simulink model "stateMachineAndGaitPlayback"  (R2016b)
settings: Solver=FixedStepAuto  StartTime=0.0  StopTime=50  FixedStep=0.002  RelTol=1e-3  AbsTol=1e-5
undefined symbols (not defined in the file or in its folder): ExoskeletonState, Leg, StepType
libraries: VariousLibrary x2, simulink x2, GaitHandler x1, StatemachineMARCH x1
settings Model: DataDictionary=ModelDictionary.sldd  Creator=Taeke  LastModifiedBy=Taeke
settings DataIOCC: SaveState=on

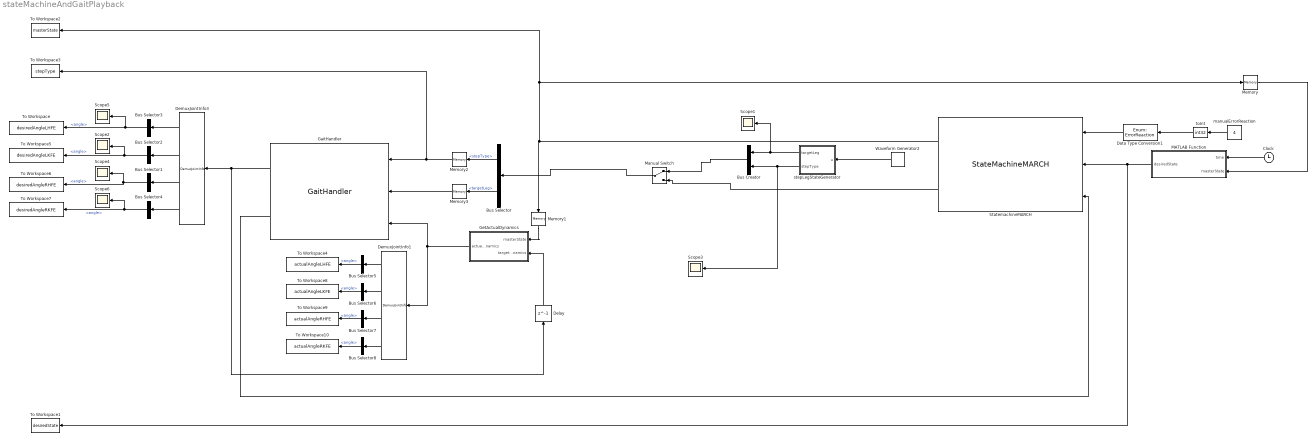
== system stateMachineAndGaitPlayback ==
  Bus Creator : BusCreator  Inputs=2  OutDataTypeStr=Bus: GaitGeneratorInput  NonVirtualBus=on
  Bus Selector : BusSelector  OutputSignals=stepType,targetLeg
  Bus Selector{1..8} (8 alike) : BusSelector  OutputSignals=angle
  Clock : Clock
  Data Type Conversion1 : DataTypeConversion  OutDataTypeStr=Enum: ErrorReaction
  Delay : Delay  DelayLength=1
  DemuxJointInfo1 : VariousLibrary/DemuxJointInfo
  DemuxJointInfo3 : VariousLibrary/DemuxJointInfo
  GaitHandler : GaitHandler/GaitHandler
  GetActualDynamics : Subsystem
  MATLAB Function : MATLAB Function  TreatAsAtomicUnit=on
  Manual Switch : ManualSwitch
  Memory : Memory  X0=ExoskeletonState.MANUAL
  Memory1 : Memory  X0=ExoskeletonState.MANUAL
  Memory2 : Memory  X0=StepType.NOSTEP
  Memory3 : Memory  X0=Leg.NONE
  Scope{1..6} (6 alike) : Scope
  StatemachineMARCH : StatemachineMARCH/StateMachineMARCH
  To Workspace : ToWorkspace  VariableName=desiredAngleLHFE  SaveFormat=Timeseries  SampleTime=-1
  To Workspace1 : ToWorkspace  VariableName=desiredState  SaveFormat=Timeseries  SampleTime=-1
  To Workspace10 : ToWorkspace  VariableName=actualAngleRKFE  SaveFormat=Timeseries  SampleTime=-1
  To Workspace2 : ToWorkspace  VariableName=masterState  SaveFormat=Timeseries  SampleTime=-1
  To Workspace3 : ToWorkspace  VariableName=stepType  SaveFormat=Timeseries  SampleTime=-1
  To Workspace4 : ToWorkspace  VariableName=actualAngleLHFE  SaveFormat=Timeseries  SampleTime=-1
  To Workspace5 : ToWorkspace  VariableName=desiredAngleLKFE  SaveFormat=Timeseries  SampleTime=-1
  To Workspace6 : ToWorkspace  VariableName=desiredAngleRHFE  SaveFormat=Timeseries  SampleTime=-1
  To Workspace7 : ToWorkspace  VariableName=desiredAngleRKFE  SaveFormat=Timeseries  SampleTime=-1
  To Workspace8 : ToWorkspace  VariableName=actualAngleLKFE  SaveFormat=Timeseries  SampleTime=-1
  To Workspace9 : ToWorkspace  VariableName=actualAngleRHFE  SaveFormat=Timeseries  SampleTime=-1
  Waveform Generator2 : simulink/Sources/Waveform Generator  OutMin=[]  OutMax=[]  OutDataTypeStr=double  SelectedSignal=1  Signals=step(1,0,1)+step(8,0,1)+step(9,0,1)+step(10.7,0,1)+step(12.4,0,1)+step(14.1,0,2)-step(15.8,0,5)+step(17,0,6)  BlockNames=MultiportSwitch_7d132669d28647b  SampleTime=-1
  manualErrorReaction : Constant  Value=4
  stepLegStateGenerator : MATLAB Function  TreatAsAtomicUnit=on
  toInt : DataTypeConversion  OutDataTypeStr=int32
  wires:
  Bus Selector/1 -> Memory2/1  "<stepType>"
  Bus Selector/2 -> Memory3/1  "<targetLeg>"
  Memory2/1 -> To Workspace3/1, GaitHandler/1
  Memory3/1 -> GaitHandler/2
  manualErrorReaction/1 -> toInt/1
  toInt/1 -> Data Type Conversion1/1
  Data Type Conversion1/1 -> StatemachineMARCH/1
  GaitHandler/2 -> StatemachineMARCH/3
  Clock/1 -> MATLAB Function/1(time)
  MATLAB Function/1(desiredState) -> StatemachineMARCH/2, To Workspace1/1
  Bus Selector1/1 -> Scope4/1, To Workspace6/1  "<angle>"
  DemuxJointInfo3/3 -> Bus Selector1/1
  Bus Selector2/1 -> Scope2/1, To Workspace5/1  "<angle>"
  DemuxJointInfo3/2 -> Bus Selector2/1
  Bus Selector3/1 -> To Workspace/1, Scope5/1  "<angle>"
  DemuxJointInfo3/1 -> Bus Selector3/1
  Bus Selector4/1 -> Scope6/1, To Workspace7/1  "<angle>"
  DemuxJointInfo3/4 -> Bus Selector4/1
  Memory/1 -> MATLAB Function/2(masterState)
  GaitHandler/1 -> Delay/1, DemuxJointInfo3/1
  DemuxJointInfo1/2 -> Bus Selector6/1
  DemuxJointInfo1/3 -> Bus Selector7/1
  DemuxJointInfo1/4 -> Bus Selector8/1
  DemuxJointInfo1/1 -> Bus Selector5/1
  Bus Selector5/1 -> To Workspace4/1  "<angle>"
  StatemachineMARCH/1 -> To Workspace2/1, Memory/1, Memory1/1
  GetActualDynamics/1(actualDynamics) -> GaitHandler/3, DemuxJointInfo1/1
  Bus Selector6/1 -> To Workspace8/1  "<angle>"
  Bus Selector7/1 -> To Workspace9/1  "<angle>"
  Bus Selector8/1 -> To Workspace10/1  "<angle>"
  Delay/1 -> GetActualDynamics/2(targetDynamics)
  Memory1/1 -> GetActualDynamics/1(masterState)
  Waveform Generator2/1 -> stepLegStateGenerator/1(u)
  Bus Creator/1 -> Manual Switch/1
  StatemachineMARCH/2 -> Manual Switch/2
  Manual Switch/1 -> Bus Selector/1
  stepLegStateGenerator/1(targetLeg) -> Scope1/1, Bus Creator/1
  stepLegStateGenerator/2(stepType) -> Scope3/1, Bus Creator/2

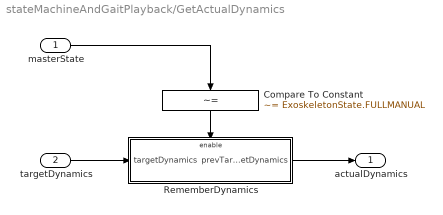
== system stateMachineAndGaitPlayback/GetActualDynamics ==
  masterState : Inport
  targetDynamics : Inport  Port=2
  Compare To Constant : simulink/Logic and Bit Operations/Compare To Constant  relop=~=  const=ExoskeletonState.FULLMANUAL  OutDataTypeStr=boolean
  RememberDynamics : Subsystem
  actualDynamics : Outport
  wires:
  Compare To Constant/1 -> RememberDynamics/Enable
  masterState/1 -> Compare To Constant/1
  targetDynamics/1 -> RememberDynamics/1(targetDynamics)
  RememberDynamics/1(prevTargetDynamics) -> actualDynamics/1

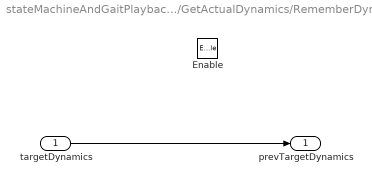
== system stateMachineAndGaitPlayback/GetActualDynamics/RememberDynamics ==
  targetDynamics : Inport
  Enable : EnablePort
  prevTargetDynamics : Outport
  wires:
  targetDynamics/1 -> prevTargetDynamics/1

== matlab function stateMachineAndGaitPlayback/MATLAB Function ==
  data: time input; desiredState output; masterState input
function desiredState = fcn(time, masterState)
desiredState = drunk_user(time, masterState);

== matlab function stateMachineAndGaitPlayback/stepLegStateGenerator ==
  data: targetLeg output; u input; stepType output
function [targetLeg, stepType]  = fcn(u)

if u==0
    stepType=StepType.HOMESIT;
    targetLeg=Leg.RIGHT;
elseif u==1
    stepType=StepType.STANDUP;
    targetLeg=Leg.RIGHT;
elseif u==2
    stepType=StepType.HOMESTAND;
    targetLeg=Leg.RIGHT;
elseif u==3
    stepType=StepType.HALFSTEPSTART;
    targetLeg=Leg.RIGHT;
elseif u==4
    stepType=StepType.FULLSTEP;
    targetLeg=Leg.LEFT;
elseif u==5
    stepType=StepType.FULLSTEP;
    targetLeg=Leg.RIGHT;
elseif u==6
    stepType=StepType.HALFSTEPSTOP;
    targetLeg=Leg.RIGHT;
elseif u==7
    stepType=StepType.HALFSTEPSTOP;
    targetLeg=Leg.LEFT;
elseif u==8
    stepType=StepType.STAIRSUPSTEP;
    targetLeg=Leg.RIGHT;
elseif u==9
    stepType=StepType.STAIRSUPSTEP;
    targetLeg=Leg.LEFT;
elseif u==10
    stepType=StepType.STAIRSDOWNSTEP;
    targetLeg=Leg.RIGHT;
elseif u==11
    stepType=StepType.STAIRSDOWNSTEP;
    targetLeg=Leg.LEFT;
else
    stepType=StepType.NOSTEP;
    targetLeg=Leg.NONE;
end
